simulink model "sensor_vs_sensorless_speed_estimation_4_2021_b"  (R2021b)
settings: Solver=VariableStepAuto  StartTime=0.0  StopTime=2  RelTol=1e-3
libraries: simulink x9, spsMosfetLib x6, slpidlib x1, spsPermanentMagnetSynchronousMachineLib x1, hdlsllib x1, dspstat3 x1, spsDCVoltageSourceLib x1, spsVoltageMeasurementLib x1, dspswit3 x1, spspowerguiLib x1
settings Model: Creator=heman  LastModifiedBy=heman
settings SolverCC: ZeroCrossAlgorithm=Adaptive
settings DebuggingCC: IgnoredZcDiagnostic=none  UnconnectedInputMsg=none  UnconnectedOutputMsg=none  UnconnectedLineMsg=none
settings ModelReferenceCC: EnableRefExpFcnMdlSchedulingChecks=off
settings RTWCC: DLArmComputeVersion=20.02.1

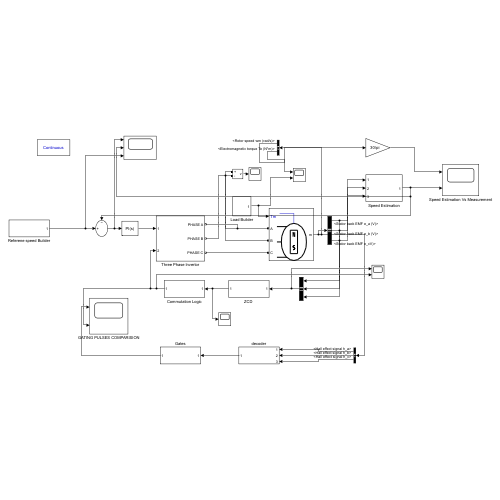
[thumbnail: Simulink's stored preview of the top-level diagram]
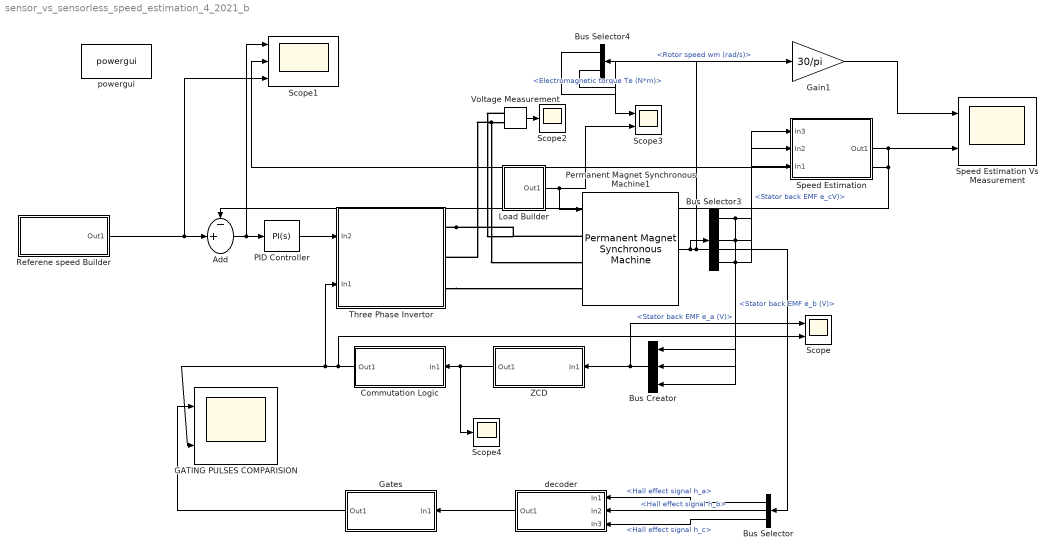
== system sensor_vs_sensorless_speed_estimation_4_2021_b ==
  Add : Sum  Inputs=-+|
  Bus Creator : BusCreator  Inputs=3
  Bus Selector : BusSelector  OutputSignals=Hall effect signal h_a,Hall effect signal h_b,Hall effect signal h_c
  Bus Selector3 : BusSelector  OutputSignals=Stator back EMF e_a (V),Stator back EMF e_b (V),Stator back EMF e_cV)
  Bus Selector4 : BusSelector  OutputSignals=Rotor speed wm (rad/s),Electromagnetic torque Te (N*m)
  Commutation Logic : Subsystem
  GATING PULSES COMPARISION : Scope  NumInputPorts=2
  Gain1 : Gain  Gain=30/pi
  Gates : Subsystem
  Load Builder : Subsystem
  PID Controller : slpidlib/PID Controller  Controller=PI  Form=Parallel  TimeDomain=Continuous-time  UseExternalTs=off  SampleTime=-1  IntegratorMethod=Forward Euler  FilterMethod=Forward Euler  ControllerParametersSource=internal  P=0.00032148  I=0.00018057  D=500  N=100  UseFilter=on  TunerSelectOption=Frequency Response Based  InitialConditionSource=internal  InitialConditionForIntegrator=0  InitialConditionForFilter=0  DifferentiatorICPrevScaledInput=0  ExternalReset=none  TrackingMode=off  Kt=1  LimitOutput=off  SatLimitsSource=internal  UpperSaturationLimit=inf  LowerSaturationLimit=-inf  LinearizeAsGain=on  AntiWindupMode=none  Kb=1  POutMin=[]  POutMax=[]  IOutMin=[]  IOutMax=[]  DOutMin=[]  DOutMax=[]  NOutMin=[]  NOutMax=[]  SumOutMin=[]  SumOutMax=[]  SaturationOutMin=[]  SaturationOutMax=[]  PParamMin=[]  PParamMax=[]  IParamMin=[]  IParamMax=[]  DParamMin=[]  DParamMax=[]  NParamMin=[]  NParamMax=[]  KbParamMin=[]  KbParamMax=[]  KtParamMin=[]  KtParamMax=[]  KbOutMin=[]  KbOutMax=[]  KtOutMin=[]  KtOutMax=[]  IntegratorOutMin=[]  IntegratorOutMax=[]  FilterOutMin=[]  FilterOutMax=[]  SumI1OutMin=[]  SumI1OutMax=[]  SumI2OutMin=[]  SumI2OutMax=[]  SumI3OutMin=[]  SumI3OutMax=[]  SumI4OutMin=[]  SumI4OutMax=[]  SumDOutMin=[]  SumDOutMax=[]  DifferentiatorOutMin=[]  DifferentiatorOutMax=[]  FilterDiffOutCoefMin=[]  FilterDiffOutCoefMax=[]  ReciprocalOutMin=[]  ReciprocalOutMax=[]  SumDenOutMin=[]  SumDenOutMax=[]  SumNumOutMin=[]  SumNumOutMax=[]  DivideOutMin=[]  DivideOutMax=[]  UdiffTsProdOutMin=[]  UdiffTsProdOutMax=[]  NTsProdOutMin=[]  NTsProdOutMax=[]  UintegralTsProdOutMin=[]  UintegralTsProdOutMax=[]  UngainTsProdOutMin=[]  UngainTsProdOutMax=[]  IntegratorContinuousStateAttributes=''  IntegratorStateMustResolveToSignalObject=off  IntegratorRTWStateStorageClass=Auto  FilterContinuousStateAttributes=''  FilterStateMustResolveToSignalObject=off  FilterRTWStateStorageClass=Auto  ParallelPVariant=InternalParameters  IdealPVariant=Disabled  IVariant=InternalParameters  DVariant=Disabled  IntegratorVariant=Continuous  SatVariant=Disabled  AWVariant=Passthrough  PCopyVariant=Disabled  TRVariant=Disabled  FdbkBlocksVariant=Forward  IdealPFdbkVariant=Disabled  SatFdbkVariant=Disabled  DerivativeFilterVariant=Disabled  NVariant=Disabled  NCopyVariant=Disabled_SignalSpec  FilterICVariant=Disabled  IntegratorICVariant=InternalICs  ExternalResetVariant=Disabled  TRSumVariant=Passthrough  SumFdbkVariant=Disabled  SumVariant=Sum_PI  TsampFilterVariant=InternalTs  TsampNgainVariant=Passthrough  TsampIntegralVariant=Disabled_SignalSpec  ExternalSaturationOutDataTypeStr=Inherit: Same as second input
  Permanent Magnet Synchronous Machine1 : spsPermanentMagnetSynchronousMachineLib/Permanent Magnet Synchronous Machine  NbPhases=3  FluxDistribution=Trapezoidal  RotorType=Round  MechanicalLoad=Torque Tm  PresetModel=No  ShowDetailedParameters=on  MeasurementBus=off  Resistance=0.7  Inductance=2.7e-3  dqInductances=[8.5e-3,8.5e-3]  La=0.000395  MachineConstant=Voltage Constant (V_peak L-L / krpm)  Flux=0.12322  VoltageCst=103.2327  TorqueCst=0.9858  Flat=120  Mechanical=[0.0027 0.0004924 4 0]  PolePairs=4  InitialConditions=[0,0, 0,0]  InitialConditions5ph=[0 0 0 0 0 0]  RefAngle=90 degrees behind phase A axis (modified Park)  IterativeDiscreteModel=Trapezoidal non iterative  TsBlock=-1  TsPowergui=0
  Referene speed Builder : Subsystem
  Scope : Scope  NumInputPorts=2
  Scope1 : Scope  NumInputPorts=3
  Scope2 : Scope
  Scope3 : Scope  NumInputPorts=2
  Scope4 : Scope
  Speed Estimation : Subsystem
  Speed Estimation Vs Measurement : Scope  NumInputPorts=2
  Three Phase Invertor : Subsystem
  Voltage Measurement : spsVoltageMeasurementLib/Voltage Measurement  PhasorSimulation=off  OutputType=Complex  PSBequivalent=0
  "ZCD " : Subsystem
  decoder : Subsystem
  powergui : spspowerguiLib/powergui  Priority=1  SimulationMode=Continuous  SampleTime=50e-6  frequency=60  Iterations=50  frequencyindice=0  Pbase=100e6  ErrMax=1e-4  UnitsV=kV  UnitsW=MW  buscounter=0  FunctionMessages=off  echomessages=off  EnableUseOfTLC=off  CurrentSourceSwitches=off  DisableSnubberDevices=off  DisableRonSwitches=off  DisableVfSwitches=off  DisplayEquations=off  AutomaticDiscreteSolvers=off  SolverType=Tustin/Backward Euler (TBE)  Interpol=off  ExternalGateDelay=off  methode=off  Ts=100  x0status=blocks  SPID=on  SwTol=0  HookPort=off  NonlinearTolerance=0  nMaxIteration=15  ContinueOnMaxIteration=off  RestoreLinks=warning  ResistiveCurrentMeasurement=off  Frange=[0:2:500]  Ylog=off  Xlog=on  ShowGrid=off  save=off  variable=ZData  structure=0  ZoomFFT=off  StartTime=0.0  cycles=1  DisplayStyle=1  fundamental=60  FreqAxis=off  MaxFrequency=1000  frequencyindicesteady=1  RmsSteady=1  display=off
  wires:
  Referene speed Builder/1(Out1) -> Scope1/3, Add/2
  Permanent Magnet Synchronous Machine1/1 -> Bus Selector/1, Bus Selector4/1, Bus Selector3/1
  Bus Creator/1 -> Scope/1, "ZCD "/1(In1)
  Bus Selector3/1 -> Bus Creator/1, Speed Estimation/3(In1)  "<Stator back EMF e_a (V)>"
  Bus Selector3/2 -> Speed Estimation/2(In2), Bus Creator/2  "<Stator back EMF e_b (V)>"
  Bus Selector3/3 -> Speed Estimation/1(In3), Bus Creator/3  "<Stator back EMF e_cV)>"
  Load Builder/1(Out1) -> Permanent Magnet Synchronous Machine1/1, Scope3/2
  Voltage Measurement/1 -> Scope2/1
  decoder/1(Out1) -> Gates/1(In1)
  Gates/1(Out1) -> GATING PULSES COMPARISION/1
  Bus Selector/1 -> decoder/1(In1)  "<Hall effect signal h_a>"
  Bus Selector/2 -> decoder/2(In2)  "<Hall effect signal h_b>"
  Bus Selector/3 -> decoder/3(In3)  "<Hall effect signal h_c>"
  "ZCD "/1(Out1) -> Commutation Logic/1(In1), Scope4/1
  Bus Selector4/1 -> Gain1/1  "<Rotor speed wm (rad/s)>"
  Gain1/1 -> Speed Estimation Vs Measurement/1
  Bus Selector4/2 -> Scope3/1  "<Electromagnetic torque Te (N*m)>"
  Speed Estimation/1(Out1) -> Add/1, Scope1/2, Speed Estimation Vs Measurement/2
  Commutation Logic/1(Out1) -> Three Phase Invertor/2(In1), GATING PULSES COMPARISION/2, Scope/2
  PID Controller/1 -> Three Phase Invertor/1(In2)
  Add/1 -> PID Controller/1, Scope1/1
  connections:
  Three Phase Invertor/RConn1 -- Permanent Magnet Synchronous Machine1/LConn1 -- Voltage Measurement/LConn1
  Voltage Measurement/LConn2 -- Permanent Magnet Synchronous Machine1/LConn2 -- Three Phase Invertor/RConn2
  Three Phase Invertor/RConn3 -- Permanent Magnet Synchronous Machine1/LConn3

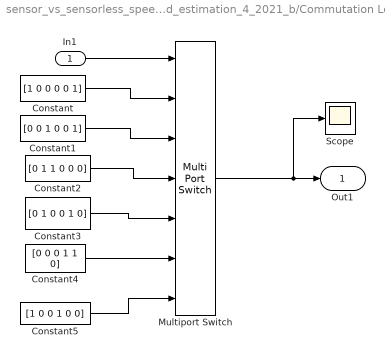
== system sensor_vs_sensorless_speed_estimation_4_2021_b/Commutation Logic ==
  In1 : Inport
  Constant : Constant  Value=[1 0 0 0 0 1]  VectorParams1D=off
  Constant1 : Constant  Value=[0 0 1 0 0 1]  VectorParams1D=off
  Constant2 : Constant  Value=[0 1 1 0 0 0]  VectorParams1D=off
  Constant3 : Constant  Value=[0 1 0 0 1 0]  VectorParams1D=off
  Constant4 : Constant  Value=[0 0 0 1 1 0]  VectorParams1D=off
  Constant5 : Constant  Value=[1 0 0 1 0 0]  VectorParams1D=off
  Multiport Switch : MultiPortSwitch  DataPortOrder=Zero-based contiguous  Inputs=6  zeroidx=on
  Scope : Scope
  Out1 : Outport
  wires:
  In1/1 -> Multiport Switch/1
  Multiport Switch/1 -> Scope/1, Out1/1
  Constant5/1 -> Multiport Switch/7
  Constant4/1 -> Multiport Switch/6
  Constant/1 -> Multiport Switch/2
  Constant1/1 -> Multiport Switch/3
  Constant2/1 -> Multiport Switch/4
  Constant3/1 -> Multiport Switch/5

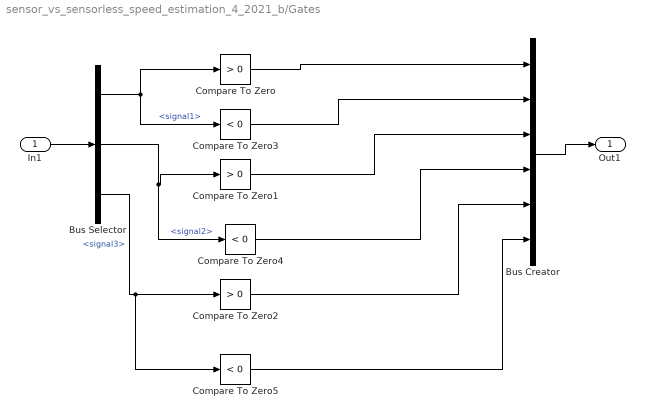
== system sensor_vs_sensorless_speed_estimation_4_2021_b/Gates ==
  In1 : Inport
  Bus Creator : BusCreator  Inputs=6
  Bus Selector : BusSelector  OutputSignals=signal1,signal2,signal3
  Compare To Zero : simulink/Logic and Bit Operations/Compare To Zero  relop=>  OutDataTypeStr=boolean
  Compare To Zero1 : simulink/Logic and Bit Operations/Compare To Zero  relop=>  OutDataTypeStr=boolean
  Compare To Zero2 : simulink/Logic and Bit Operations/Compare To Zero  relop=>  OutDataTypeStr=boolean
  Compare To Zero3 : simulink/Logic and Bit Operations/Compare To Zero  relop=<  OutDataTypeStr=boolean
  Compare To Zero4 : simulink/Logic and Bit Operations/Compare To Zero  relop=<  OutDataTypeStr=boolean
  Compare To Zero5 : simulink/Logic and Bit Operations/Compare To Zero  relop=<  OutDataTypeStr=boolean
  Out1 : Outport
  wires:
  In1/1 -> Bus Selector/1
  Compare To Zero/1 -> Bus Creator/1
  Compare To Zero1/1 -> Bus Creator/3
  Bus Creator/1 -> Out1/1
  Compare To Zero2/1 -> Bus Creator/5
  Compare To Zero3/1 -> Bus Creator/2
  Bus Selector/1 -> Compare To Zero3/1, Compare To Zero/1  "<signal1>"
  Bus Selector/2 -> Compare To Zero4/1, Compare To Zero1/1  "<signal2>"
  Compare To Zero4/1 -> Bus Creator/4
  Compare To Zero5/1 -> Bus Creator/6
  Bus Selector/3 -> Compare To Zero5/1, Compare To Zero2/1  "<signal3>"

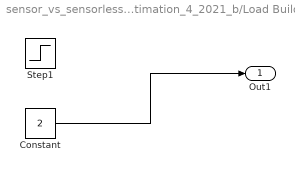
== system sensor_vs_sensorless_speed_estimation_4_2021_b/Load Builder ==
  Constant : Constant  Value=2
  Step1 : Step  Time=0  After=5  SampleTime=0
  Out1 : Outport
  wires:
  Constant/1 -> Out1/1

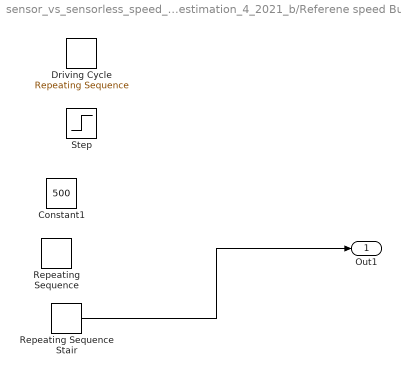
== system sensor_vs_sensorless_speed_estimation_4_2021_b/Referene speed Builder ==
  Constant1 : Constant  Value=500
  Driving Cycle : simulink/Sources/Repeating Sequence  rep_seq_t=[0 1 2 3 4 5 6 7 8 9 10 11 11.0001 12 13]*5/13  rep_seq_y=[0 0 10 10 0 0 20 20 0 0 35 35 25 25 0]*10
  Repeating Sequence : simulink/Sources/Repeating Sequence  rep_seq_t=[0 2]*2  rep_seq_y=[300 2500]
  Repeating Sequence Stair : simulink/Sources/Repeating Sequence Stair  OutValues=[250 500 1000 1500 1800]  tsamp=0.25  OutMin=[]  OutMax=[]  OutDataTypeStr=double  OutputDataTypeScalingMode=double  OutDataType=fixdt(0,8)  ConRadixGroup=Best Precision: Vector-wise  OutScaling=2^-12
  Step : Step  Time=0  After=2000  SampleTime=0
  Out1 : Outport
  wires:
  Repeating Sequence Stair/1 -> Out1/1

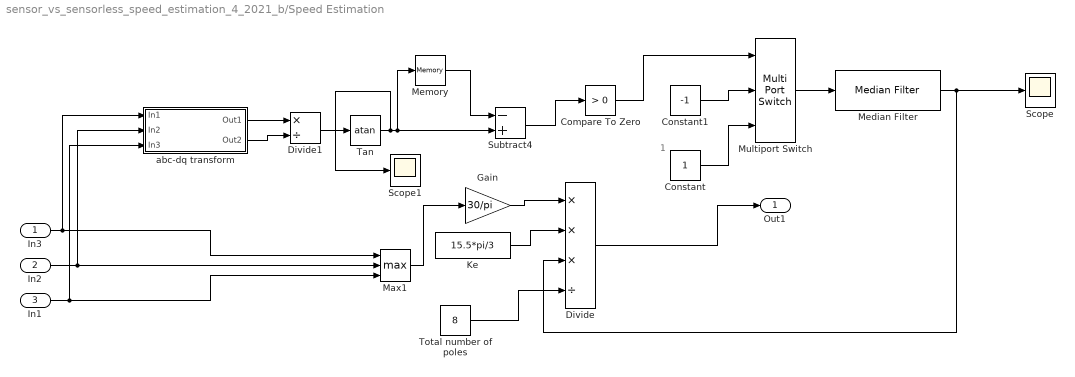
== system sensor_vs_sensorless_speed_estimation_4_2021_b/Speed Estimation ==
  note: 1
  In3 : Inport
  In2 : Inport  Port=2
  In1 : Inport  Port=3
  Compare To Zero : hdlsllib/Logic and Bit Operations/Compare To Zero  relop=>  OutDataTypeStr=uint8
  Constant : Constant
  Constant1 : Constant  Value=-1
  Divide : Product  Inputs=***/
  Divide1 : Product  Inputs=*/
  Gain : Gain  Gain=30/pi
  Ke : Constant  Value=15.5*pi/3
  Max1 : MinMax  Function=max  Inputs=3
  Median Filter : dspstat3/Median Filter  WindowLength=5  SimulateUsing=Interpreted execution
  Memory : Memory
  Multiport Switch : MultiPortSwitch  DataPortOrder=Zero-based contiguous  Inputs=2  zeroidx=on
  Scope : Scope
  Scope1 : Scope
  Subtract4 : Sum  Inputs=-+
  Tan : Trigonometry  Operator=atan
  Total number of poles : Constant  Value=8
  abc-dq transform : Subsystem
  Out1 : Outport
  wires:
  Max1/1 -> Gain/1
  Divide/1 -> Out1/1
  Gain/1 -> Divide/1
  Ke/1 -> Divide/2
  In1/1 -> abc-dq transform/3(In3), Max1/3
  In3/1 -> abc-dq transform/1(In1), Max1/1
  In2/1 -> abc-dq transform/2(In2), Max1/2
  Divide1/1 -> Tan/1
  Tan/1 -> Scope1/1, Subtract4/2, Memory/1
  Memory/1 -> Subtract4/1
  Subtract4/1 -> Compare To Zero/1
  Compare To Zero/1 -> Multiport Switch/1
  Constant1/1 -> Multiport Switch/2
  Constant/1 -> Multiport Switch/3
  Multiport Switch/1 -> Median Filter/1
  Total number of poles/1 -> Divide/4
  abc-dq transform/1(Out1) -> Divide1/1
  abc-dq transform/2(Out2) -> Divide1/2
  Median Filter/1 -> Divide/3, Scope/1

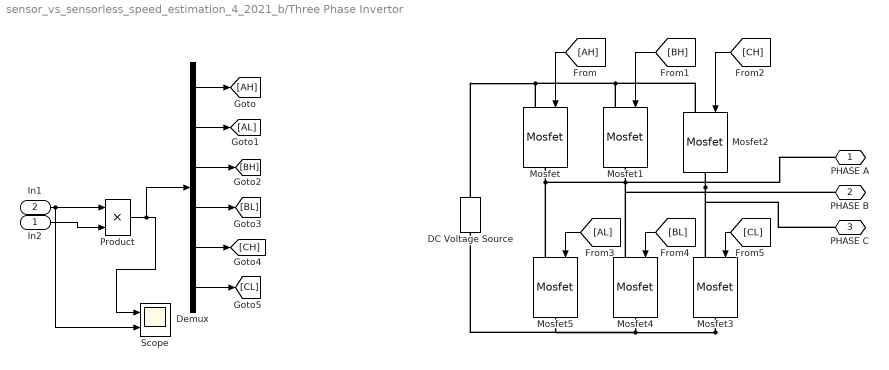
== system sensor_vs_sensorless_speed_estimation_4_2021_b/Three Phase Invertor ==
  In2 : Inport
  In1 : Inport  Port=2
  DC Voltage Source : spsDCVoltageSourceLib/DC Voltage Source  Amplitude=150  Measurements=None
  Demux : Demux  Outputs=6
  Mosfet{,1..5} (6 alike) : spsMosfetLib/Mosfet  Ron=1e-3  Lon=0  Rd=0.01  Vfd=0  IC=0  Rs=1e5  Cs=inf  Measurements=off
  Product : Product
  Scope : Scope  NumInputPorts=2
  PHASE A : PMIOPort  Side=Right
  PHASE B : PMIOPort  Port=2  Side=Right
  PHASE C : PMIOPort  Port=3  Side=Right
  wires:
  [AH] -> Mosfet/1
  [CH] -> Mosfet2/1
  [BH] -> Mosfet1/1
  [AL] -> Mosfet5/1
  [BL] -> Mosfet4/1
  [CL] -> Mosfet3/1
  Demux/1 -> [AH]
  Demux/2 -> [AL]
  Demux/3 -> [BH]
  Demux/4 -> [BL]
  Demux/5 -> [CH]
  Demux/6 -> [CL]
  In1/1 -> Scope/2, Product/1
  In2/1 -> Product/2
  Product/1 -> Demux/1, Scope/1
  connections:
  Mosfet3/RConn1 -- DC Voltage Source/LConn1 -- Mosfet5/RConn1 -- Mosfet4/RConn1
  Mosfet2/RConn1 -- Mosfet3/LConn1 -- PHASE C/RConn1
  Mosfet1/RConn1 -- PHASE B/RConn1 -- Mosfet4/LConn1
  Mosfet1/LConn1 -- Mosfet2/LConn1 -- DC Voltage Source/RConn1 -- Mosfet/LConn1
  Mosfet/RConn1 -- Mosfet5/LConn1 -- PHASE A/RConn1

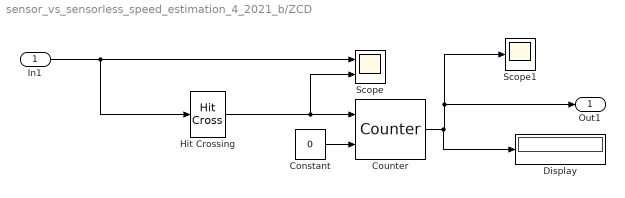
== system sensor_vs_sensorless_speed_estimation_4_2021_b/ZCD  ==
  In1 : Inport
  Constant : Constant  Value=0
  Counter : dspswit3/Counter  Direction=Up  CountEvent=Rising edge  CounterSize=User defined  MaxCount=5  InitialCount=0  Output=Count  HitValue=32  ResetInput=on  SamplesPerFrame=1  Ts=1  CntDtype=double  HitDtype=Logical
  Display : Display
  Hit Crossing : HitCross
  Scope : Scope  NumInputPorts=2
  Scope1 : Scope
  Out1 : Outport
  wires:
  In1/1 -> Scope/1, Hit Crossing/1
  Hit Crossing/1 -> Scope/2, Counter/1
  Constant/1 -> Counter/2
  Counter/1 -> Scope1/1, Out1/1, Display/1

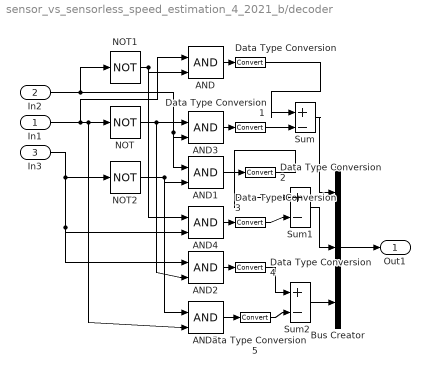
== system sensor_vs_sensorless_speed_estimation_4_2021_b/decoder ==
  In1 : Inport
  In2 : Inport  Port=2
  In3 : Inport  Port=3
  AND{,1..5} (6 alike) : Logic  IconShape=distinctive  AllPortsSameDT=off  OutDataTypeStr=boolean
  Bus Creator : BusCreator  Inputs=3
  Data Type Conversion{,1..5} (6 alike) : DataTypeConversion
  NOT : Logic  Operator=NOT  IconShape=distinctive  AllPortsSameDT=off  OutDataTypeStr=boolean
  NOT1 : Logic  Operator=NOT  IconShape=distinctive  AllPortsSameDT=off  OutDataTypeStr=boolean
  NOT2 : Logic  Operator=NOT  IconShape=distinctive  AllPortsSameDT=off  OutDataTypeStr=boolean
  Sum : Sum  Inputs=|+-
  Sum1 : Sum  Inputs=|+-
  Sum2 : Sum  Inputs=|+-
  Out1 : Outport
  wires:
  In2/1 -> AND1/1, AND3/2, NOT1/1
  In1/1 -> AND5/2, NOT/1, AND/1
  NOT/1 -> AND3/1, AND2/2
  In3/1 -> AND4/2, AND2/1, NOT2/1
  NOT1/1 -> AND/2, AND4/1
  NOT2/1 -> AND5/1, AND1/2
  Sum/1 -> Bus Creator/1
  Sum1/1 -> Bus Creator/2
  Sum2/1 -> Bus Creator/3
  Bus Creator/1 -> Out1/1
  AND/1 -> Data Type Conversion/1
  AND3/1 -> Data Type Conversion1/1
  Data Type Conversion1/1 -> Sum/2
  Data Type Conversion/1 -> Sum/1
  AND1/1 -> Data Type Conversion2/1
  Data Type Conversion2/1 -> Sum1/1
  AND4/1 -> Data Type Conversion3/1
  Data Type Conversion3/1 -> Sum1/2
  AND2/1 -> Data Type Conversion4/1
  AND5/1 -> Data Type Conversion5/1
  Data Type Conversion5/1 -> Sum2/2
  Data Type Conversion4/1 -> Sum2/1

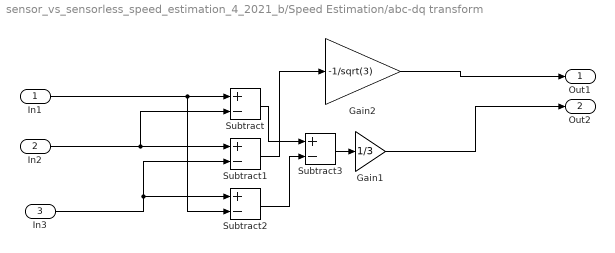
== system sensor_vs_sensorless_speed_estimation_4_2021_b/Speed Estimation/abc-dq transform ==
  In1 : Inport
  In2 : Inport  Port=2
  In3 : Inport  Port=3
  Gain1 : Gain  Gain=1/3
  Gain2 : Gain  Gain=-1/sqrt(3)
  Subtract{,1..3} (4 alike) : Sum  Inputs=+-
  Out1 : Outport
  Out2 : Outport  Port=2
  wires:
  Subtract/1 -> Subtract3/1
  Gain2/1 -> Out1/1
  Subtract2/1 -> Subtract3/2
  Subtract1/1 -> Gain2/1
  Subtract3/1 -> Gain1/1
  In1/1 -> Subtract2/2, Subtract/1
  In2/1 -> Subtract1/1, Subtract/2
  In3/1 -> Subtract2/1, Subtract1/2
  Gain1/1 -> Out2/1
